simulink model "verify_Storage_Type_1_mdl"  (R2016b)
settings: Solver=ode45  StartTime=time(1)  StopTime=time(end)  MaxStep=time(2)-time(1)  RelTol=1e-3  EnableMultiTasking=on
InitFcn:
  | load('data_EN12977_sequence_V')
libraries: carnot x11
settings Model: Creator=drhf  LastModifiedBy=drhf
settings DataIOCC: SaveFormat=Array  SignalLoggingSaveFormat=ModelDataLogs
settings OptimizationCC: ExpressionDepthLimit=2147483647  LifeSpan=inf
settings DebuggingCC: UnderspecifiedInitializationDetection=Classic  MergeDetectMultiDrivingBlocksExec=none  SolverPrmCheckMsg=warning  FcnCallInpInsideContextMsg=warning  StateNameClashWarn=warning  SFUnexpectedBacktrackingDiag=warning  SFNoUnconditionalDefaultTransitionDiag=warning  SFExecutionAtInitializationDiag=none
settings HardwareCC: ProdBitPerPointer=32  ProdBitPerSizeT=32  ProdBitPerPtrDiffT=32  ProdLargestAtomicFloat=None  ProdIntDivRoundTo=Undefined  ProdEndianess=Unspecified  ProdWordSize=32  ProdHWDeviceType=32-bit Generic
settings ModelReferenceCC: PropagateSignalLabelsOutOfModel=off
settings GRTTargetCC: TargetLangStandard=C89/C90 (ANSI)  GeneratePreprocessorConditionals=Disable all  CombineOutputUpdateFcns=off  GRTInterface=on
settings ConfigComp: CovMetricSettings=dw  CovHtmlReporting=on  CovSaveCumulativeToWorkspaceVar=on  CovSaveSingleToWorkspaceVar=on  CovExternalEMLEnable=off

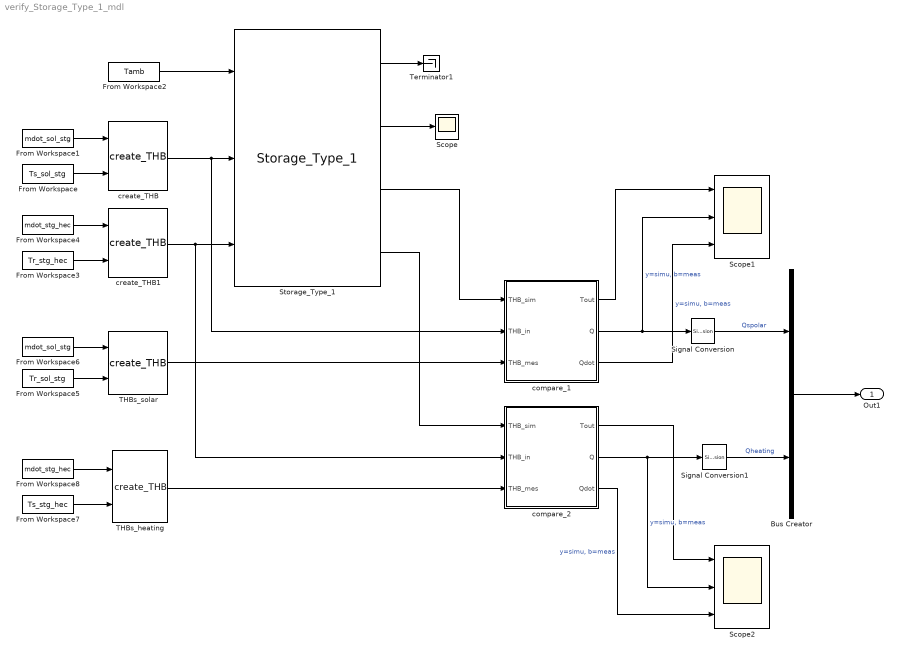
== system verify_Storage_Type_1_mdl ==
  Bus Creator : BusCreator  Inputs=2
  From Workspace : FromWorkspace  VariableName=Ts_sol_stg  SampleTime=0
  From Workspace1 : FromWorkspace  VariableName=mdot_sol_stg  SampleTime=0
  From Workspace2 : FromWorkspace  VariableName=Tamb  SampleTime=0
  From Workspace3 : FromWorkspace  VariableName=Tr_stg_hec  SampleTime=0
  From Workspace4 : FromWorkspace  VariableName=mdot_stg_hec  SampleTime=0
  From Workspace5 : FromWorkspace  VariableName=Tr_sol_stg  SampleTime=0
  From Workspace6 : FromWorkspace  VariableName=mdot_sol_stg  SampleTime=0
  From Workspace7 : FromWorkspace  VariableName=Ts_stg_hec  SampleTime=0
  From Workspace8 : FromWorkspace  VariableName=mdot_stg_hec  SampleTime=0
  Scope : Scope
  Scope1 : Scope  NumInputPorts=3
  Scope2 : Scope  NumInputPorts=3
  Signal Conversion : SignalConversion  OverrideOpt=off
  Signal Conversion1 : SignalConversion  OverrideOpt=off
  Storage_Type_1 : carnot/Storage/Thermal/Storage_Type_1  uloss=1.4  ubot=1.4  utop=1.4  cond=1.2  volume=0.220  dia=0.53  pos=standing cylinder  h_in_chg=0.62  h_out_chg=0  dplin_chg=0  dpqua_chg=0  h_in=0.1  h_out=1  dplin=0  dpqua=0  t0=interp1(1:10, Tstg(1, 2:end), 10:-9/99:1)  nodes=100  mpoints=20
  THBs_heating : carnot/Source/Simple/create_THB  p=1e5  fluid=Water  mix=0  dia=0.02  mID=No Pressure Drop
  THBs_solar : carnot/Source/Simple/create_THB  p=1e5  fluid=Water  mix=0  dia=0.02  mID=No Pressure Drop
  Terminator1 : Terminator
  compare_1 : Subsystem
  compare_2 : Subsystem
  create_THB : carnot/Source/Simple/create_THB  p=1e5  fluid=Water  mix=0  dia=0.02  mID=No Pressure Drop
  create_THB1 : carnot/Source/Simple/create_THB  p=1e5  fluid=Water  mix=0  dia=0.02  mID=No Pressure Drop
  Out1 : Outport
  wires:
  From Workspace2/1 -> Storage_Type_1/1
  create_THB/1 -> compare_1/2(THB_in), Storage_Type_1/2
  create_THB1/1 -> compare_2/2(THB_in), Storage_Type_1/3
  Storage_Type_1/2 -> Scope/1
  Storage_Type_1/3 -> compare_1/1(THB_sim)
  Storage_Type_1/4 -> compare_2/1(THB_sim)
  Bus Creator/1 -> Out1/1
  From Workspace/1 -> create_THB/2
  From Workspace1/1 -> create_THB/1
  From Workspace4/1 -> create_THB1/1
  From Workspace3/1 -> create_THB1/2
  Storage_Type_1/1 -> Terminator1/1
  From Workspace6/1 -> THBs_solar/1
  From Workspace5/1 -> THBs_solar/2
  From Workspace8/1 -> THBs_heating/1
  From Workspace7/1 -> THBs_heating/2
  THBs_solar/1 -> compare_1/3(THB_mes)
  THBs_heating/1 -> compare_2/3(THB_mes)
  compare_1/1(Tout) -> Scope1/1
  compare_1/2(Q) -> Scope1/2, Signal Conversion/1  "y=simu, b=meas"
  compare_1/3(Qdot) -> Scope1/3  "y=simu, b=meas"
  compare_2/3(Qdot) -> Scope2/3  "y=simu, b=meas"
  compare_2/2(Q) -> Scope2/2, Signal Conversion1/1  "y=simu, b=meas"
  compare_2/1(Tout) -> Scope2/1
  Signal Conversion/1 -> Bus Creator/1  "Qspolar"
  Signal Conversion1/1 -> Bus Creator/2  "Qheating"

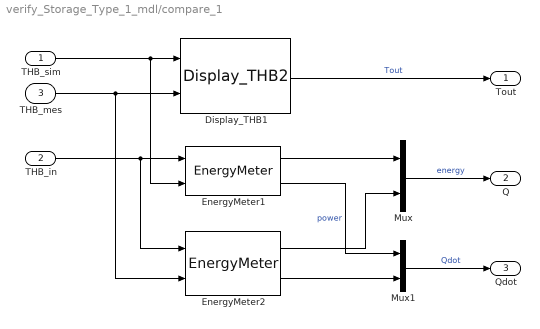
== system verify_Storage_Type_1_mdl/compare_1 ==
  THB_sim : Inport
  THB_in : Inport  Port=2
  THB_mes : Inport  Port=3
  Display_THB1 : carnot/Outputs/Display_THB2  t=on  m=off  p=off  id=off  mix=off  d=off
  EnergyMeter1 : carnot/Control/EnergyMeter
  EnergyMeter2 : carnot/Control/EnergyMeter
  Mux : Mux  Inputs=2
  Mux1 : Mux  Inputs=2
  Tout : Outport
  Q : Outport  Port=2
  Qdot : Outport  Port=3
  wires:
  THB_sim/1 -> EnergyMeter1/2, Display_THB1/1
  THB_mes/1 -> EnergyMeter2/2, Display_THB1/2
  EnergyMeter1/1 -> Mux/1
  Display_THB1/1 -> Tout/1  "Tout"
  Mux/1 -> Q/1  "energy"
  EnergyMeter1/2 -> Mux1/1  "power"
  Mux1/1 -> Qdot/1  "Qdot"
  THB_in/1 -> EnergyMeter2/1, EnergyMeter1/1
  EnergyMeter2/1 -> Mux/2
  EnergyMeter2/2 -> Mux1/2

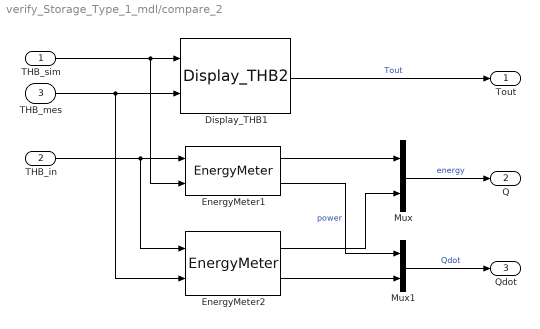
== system verify_Storage_Type_1_mdl/compare_2 ==
  THB_sim : Inport
  THB_in : Inport  Port=2
  THB_mes : Inport  Port=3
  Display_THB1 : carnot/Outputs/Display_THB2  t=on  m=off  p=off  id=off  mix=off  d=off
  EnergyMeter1 : carnot/Control/EnergyMeter
  EnergyMeter2 : carnot/Control/EnergyMeter
  Mux : Mux  Inputs=2
  Mux1 : Mux  Inputs=2
  Tout : Outport
  Q : Outport  Port=2
  Qdot : Outport  Port=3
  wires:
  EnergyMeter2/2 -> Mux1/2
  EnergyMeter2/1 -> Mux/2
  THB_in/1 -> EnergyMeter1/1, EnergyMeter2/1
  Mux1/1 -> Qdot/1  "Qdot"
  EnergyMeter1/2 -> Mux1/1  "power"
  Mux/1 -> Q/1  "energy"
  Display_THB1/1 -> Tout/1  "Tout"
  EnergyMeter1/1 -> Mux/1
  THB_mes/1 -> Display_THB1/2, EnergyMeter2/2
  THB_sim/1 -> Display_THB1/1, EnergyMeter1/2
